simulink model "q5_hw4"  (R2020a)
settings: Solver=VariableStepAuto  StartTime=0.0  StopTime=50  RelTol=1e-3
settings Model: Creator=rahulswa  LastModifiedBy=rahulswa

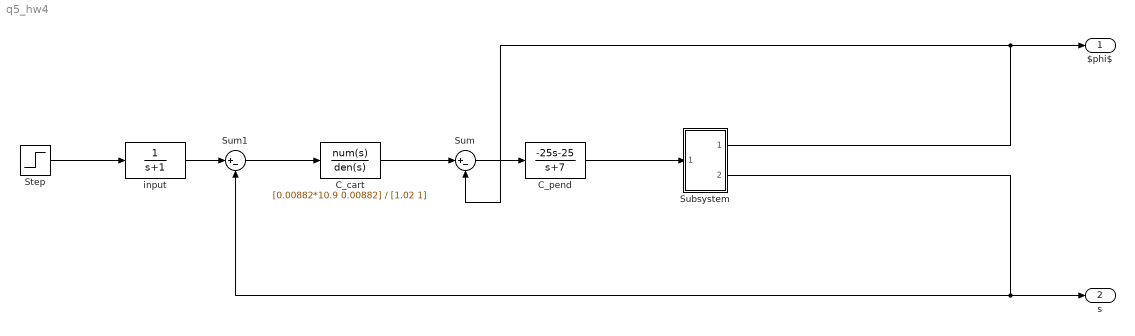
== system q5_hw4 ==
  C_cart : TransferFcn  Numerator=[0.00882*10.9 0.00882]  Denominator=[1.02 1]
  C_pend : TransferFcn  Numerator=[-25 -25]  Denominator=[1 7]
  Step : Step  After=10  SampleTime=0
  Subsystem : Subsystem
  Sum : Sum  Inputs=|+-
  Sum1 : Sum  Inputs=|+-
  input : TransferFcn  Denominator=[1 1]
  $phi$ : Outport
  s : Outport  Port=2
  wires:
  C_pend/1 -> Subsystem/1(In1)
  Subsystem/1(Out1) -> Sum/2, $phi$/1
  Sum1/1 -> C_cart/1
  C_cart/1 -> Sum/1
  Sum/1 -> C_pend/1
  Subsystem/2(Out2) -> Sum1/2, s/1
  input/1 -> Sum1/1
  Step/1 -> input/1

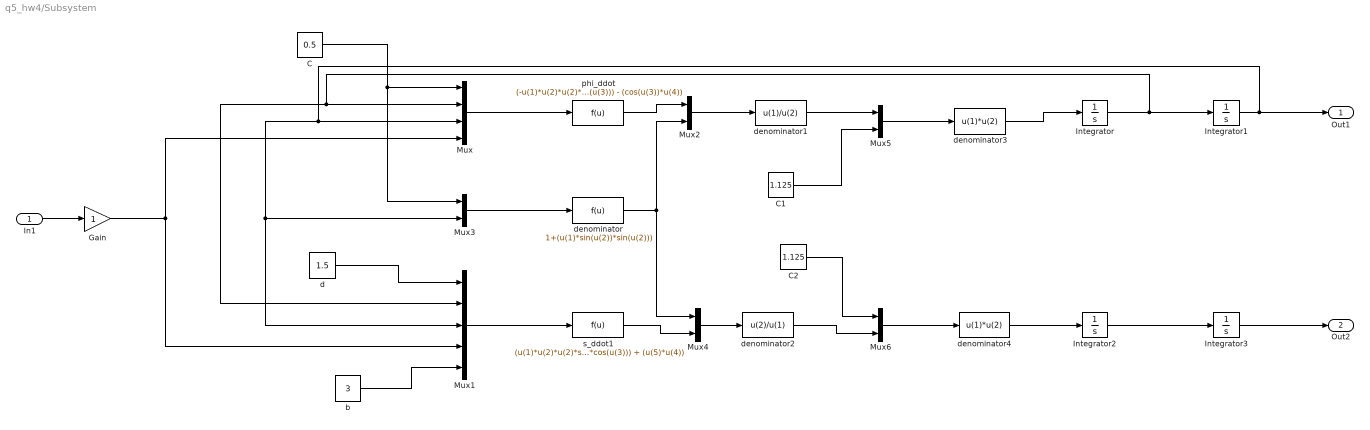
== system q5_hw4/Subsystem ==
  In1 : Inport
  C : Constant  Value=0.5
  C1 : Constant  Value=1.125
  C2 : Constant  Value=1.125
  Gain : Gain
  Integrator{,1..3} (4 alike) : Integrator
  Mux : Mux
  Mux1 : Mux  Inputs=5
  Mux{2..6} (5 alike) : Mux  Inputs=2
  b : Constant  Value=3
  d : Constant  Value=1.5
  denominator : Fcn  Expr=1+(u(1)*sin(u(2))*sin(u(2)))
  denominator1 : Fcn  Expr=u(1)/u(2)
  denominator2 : Fcn  Expr=u(2)/u(1)
  denominator3 : Fcn  Expr=u(1)*u(2)
  denominator4 : Fcn  Expr=u(1)*u(2)
  phi_ddot : Fcn  Expr=(-u(1)*u(2)*u(2)*sin(u(3))*cos(u(3))) + (sin(u(3))) - (cos(u(3))*u(4))
  s_ddot1 : Fcn  Expr=(u(1)*u(2)*u(2)*sin(u(3))) - (sin(u(3))*cos(u(3))) + (u(5)*u(4))
  Out1 : Outport
  Out2 : Outport  Port=2
  wires:
  Mux3/1 -> denominator/1
  denominator/1 -> Mux4/1, Mux2/2
  Integrator1/1 -> Out1/1, Mux1/3, Mux3/2, Mux/3
  phi_ddot/1 -> Mux2/1
  Mux/1 -> phi_ddot/1
  Mux2/1 -> denominator1/1
  C/1 -> Mux3/1, Mux/1
  Integrator3/1 -> Out2/1
  Integrator/1 -> Mux1/2, Mux/2, Integrator1/1
  Mux1/1 -> s_ddot1/1
  d/1 -> Mux1/1
  b/1 -> Mux1/5
  Integrator2/1 -> Integrator3/1
  s_ddot1/1 -> Mux4/2
  Mux4/1 -> denominator2/1
  denominator1/1 -> Mux5/1
  C1/1 -> Mux5/2
  denominator2/1 -> Mux6/2
  C2/1 -> Mux6/1
  Mux5/1 -> denominator3/1
  denominator3/1 -> Integrator/1
  Mux6/1 -> denominator4/1
  denominator4/1 -> Integrator2/1
  Gain/1 -> Mux/4, Mux1/4
  In1/1 -> Gain/1
